simulink model "gm_rampa_vnl"  (R2017a)
settings: Solver=FixedStepDiscrete  StartTime=0.0  StopTime=10.0  FixedStep=0.001  MaxStep=1e-4  RelTol=1e-3
undefined symbols (not defined in the file or in its folder): N
libraries: simulink x2
settings Model: Creator=Windows  LastModifiedBy=Windows
settings DataIOCC: LimitDataPoints=on  SaveOutput=off  SaveTime=off
settings OptimizationCC: BlockReduction=off  ConditionallyExecuteInputs=off  DefaultParameterBehavior=Inlined  LifeSpan=inf
settings DebuggingCC: AlgebraicLoopMsg=error  InheritedTsInSrcMsg=none  SingleTaskRateTransMsg=error  AllowSymbolicDim=off  StrictBusMsg=ErrorOnBusTreatedAsVector  SFUnexpectedBacktrackingDiag=warning  SFNoUnconditionalDefaultTransitionDiag=warning  SFExecutionAtInitializationDiag=none
settings HardwareCC: ProdBitPerPointer=32  ProdBitPerSizeT=32  ProdBitPerPtrDiffT=32  ProdLargestAtomicFloat=None  ProdIntDivRoundTo=Undefined  ProdEndianess=Unspecified  ProdWordSize=32  ProdHWDeviceType=ASIC/FPGA->ASIC/FPGA  TargetBitPerPointer=64  TargetBitPerSizeT=64  TargetBitPerPtrDiffT=64  TargetLongLongMode=on  TargetIntDivRoundTo=Zero  TargetEndianess=LittleEndian  TargetWordSize=64  TargetHWDeviceType=MATLAB Host  ProdEqTarget=off
settings GRTTargetCC: TargetLangStandard=C89/C90 (ANSI)  GeneratePreprocessorConditionals=Disable all
settings ConfigComp: CovScope=ReferencedModels  CovMetricSettings=dw  CovHtmlReporting=on  CovSaveCumulativeToWorkspaceVar=on  CovSaveSingleToWorkspaceVar=on  CovExternalEMLEnable=off  CovSFcnEnable=off

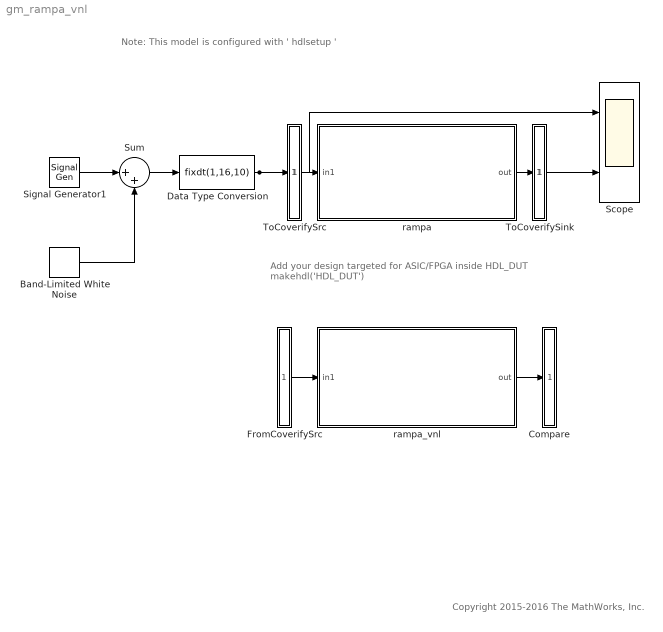
== system gm_rampa_vnl ==
  note: Note: This model is configured with ' hdlsetup '
  note: Add your design targeted for ASIC/FPGA inside HDL_DUT
      | makehdl('HDL_DUT')
  note: Copyright 2015-2016 The MathWorks, Inc.
  Band-Limited White Noise : simulink/Sources/Band-Limited White Noise  Cov=[0.001]  Ts=0.001  seed=[23341]
  Compare : Subsystem
      mask Display: disp('')
  Data Type Conversion : DataTypeConversion  OutDataTypeStr=fixdt(1,16,10)
  FromCoverifySrc : Subsystem
      mask Display: disp('')
  Scope : Scope  NumInputPorts=2
  Signal Generator1 : SignalGenerator  Frequency=2000
  Sum : Sum  Inputs=|++
  ToCoverifySink : Subsystem
      mask Display: disp('')
  ToCoverifySrc : Subsystem
      mask Display: disp('')
  rampa : Subsystem
  rampa_vnl : Subsystem
  wires:
  Data Type Conversion/1 -> Scope/1, ToCoverifySrc/1(in1)
  Signal Generator1/1 -> Sum/1
  Sum/1 -> Data Type Conversion/1
  Band-Limited White Noise/1 -> Sum/2
  ToCoverifySrc/1(out1) -> rampa/1(in1)
  rampa/1(out) -> ToCoverifySink/1(in1)
  ToCoverifySink/1(out1) -> Scope/2
  FromCoverifySrc/1(out1) -> rampa_vnl/1(in1)
  rampa_vnl/1(out) -> Compare/1(in1)

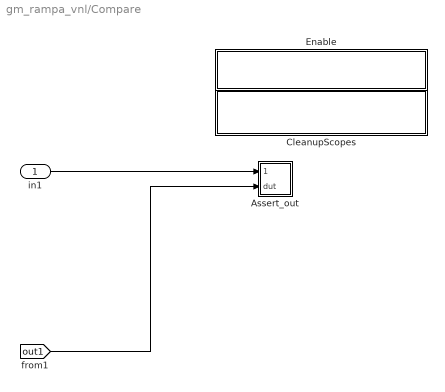
== system gm_rampa_vnl/Compare ==
  in1 : Inport
  Assert_out : Subsystem
  CleanupScopes : Subsystem
      settings: OpenFcn=|
      | blkName = gcb; %self block
      | idx = regexp(blkName, '/CleanupScopes$', 'once');
      | blkParent = blkName(1:idx-1);
      | blks=find_system(blkParent, 'LookUnderMasks', 'all','blocktype', 'Scope');
      | for itr = 1:length(blks)
      | 	 hScopeCfg = get_param(blks{itr},'ScopeConfiguration');
      | 	 hScopeCfg.Visible = ~ hScopeCfg.Visible;
      | end
      | drawnow;
      mask Display: fprintf(message('hdlcoder:cosim:vnl_dblclick').getString());
  Enable : Subsystem
      settings: OpenFcn=|
      | blkName = gcb;
      | idx = regexp(blkName, '/Enable$', 'once');
      | blkParent = blkName(1:idx-1);
      | blks=find_system(blkParent, 'LookUnderMasks', 'all','blocktype', 'Assertion');
      | e = get_param(blks{1}, 'Enabled');
      | if strcmp(e, 'on'), f= 'off';, else, f = 'on';, end
      | for ii=1:length(blks), set_param(blks{ii}, 'Enabled', f);, end
      | set_param(gcb, 'MaskDisplay',['fprintf(message(''hdlcoder:cosim:vnl_dblclick_assertions'',','''',upper(e),'''',').getString())']);
      mask Display: fprintf(message('hdlcoder:cosim:vnl_dblclick_assertions','OFF').getString());
  wires:
  in1/1 -> Assert_out/1(cosim)
  [out1] -> Assert_out/2(dut)

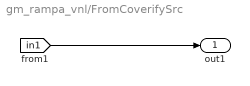
== system gm_rampa_vnl/FromCoverifySrc ==
  out1 : Outport
  wires:
  [in1] -> out1/1

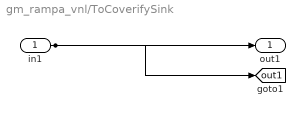
== system gm_rampa_vnl/ToCoverifySink ==
  in1 : Inport
  out1 : Outport
  tag scope: out1=global
  wires:
  in1/1 -> out1/1, [out1]

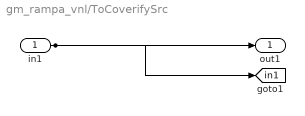
== system gm_rampa_vnl/ToCoverifySrc ==
  in1 : Inport
  out1 : Outport
  tag scope: in1=global
  wires:
  in1/1 -> out1/1, [in1]

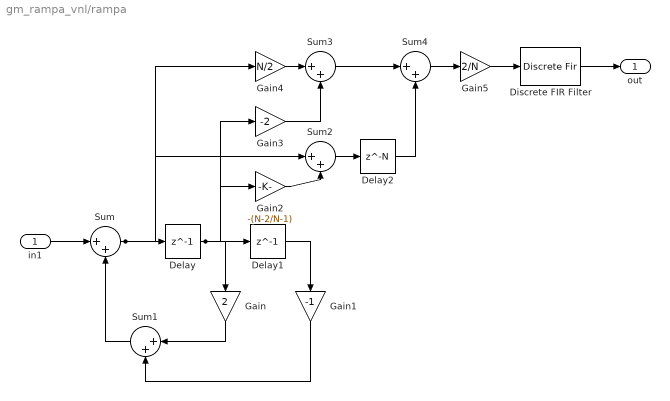
== system gm_rampa_vnl/rampa ==
  in1 : Inport  OutDataTypeStr=fixdt(1, 16, 10)  SampleTime=0
  Delay : Delay  DelayLength=1
  Delay1 : Delay  DelayLength=1
  Delay2 : Delay  DelayLength=N
  Discrete FIR Filter : DiscreteFir  Coefficients=[0.1095 0.1047 0.1000 0.0952 0.0904 0.0857 0.0809 0.0761 0.0714 0.0666 0.0619 0.0571 0.0523 0.0476 0.0428 0.0380 0.0333 0.0285 0.0238 0.0190 0.0142 0.0095 0.0047 0 -0.0047 -0.0095 -0.0142 -0.0190 -0.0238 -0.0285 -0.0333 -0.0380 -0.0428 -0.0476 -0.0523]  CoefDataTypeStr=fixdt(1,16,10)  ProductDataTypeStr=fixdt(1,16,10)  AccumDataTypeStr=fixdt(1,16,10)  OutDataTypeStr=fixdt(1,16,10)
  Gain : Gain  Gain=2
  Gain1 : Gain  Gain=-1
  Gain2 : Gain  Gain=-(N-2/N-1)
  Gain3 : Gain  Gain=-2
  Gain4 : Gain  Gain=N/2
  Gain5 : Gain  Gain=2/N
  Sum{,1..4} (5 alike) : Sum  Inputs=|++  AccumDataTypeStr=fixdt(1,16,10)  OutDataTypeStr=fixdt(1,16,10)
  out : Outport  OutDataTypeStr=fixdt(1,16,10)
  wires:
  Sum4/1 -> Gain5/1
  Sum3/1 -> Sum4/1
  Sum2/1 -> Delay2/1
  Sum1/1 -> Sum/2
  Sum/1 -> Delay/1, Gain4/1, Sum2/1
  Gain5/1 -> Discrete FIR Filter/1
  Gain4/1 -> Sum3/1
  Gain3/1 -> Sum3/2
  Gain2/1 -> Sum2/2
  Gain1/1 -> Sum1/2
  Gain/1 -> Sum1/1
  Discrete FIR Filter/1 -> out/1
  Delay2/1 -> Sum4/2
  Delay1/1 -> Gain1/1
  Delay/1 -> Delay1/1, Gain/1, Gain2/1, Gain3/1
  in1/1 -> Sum/1

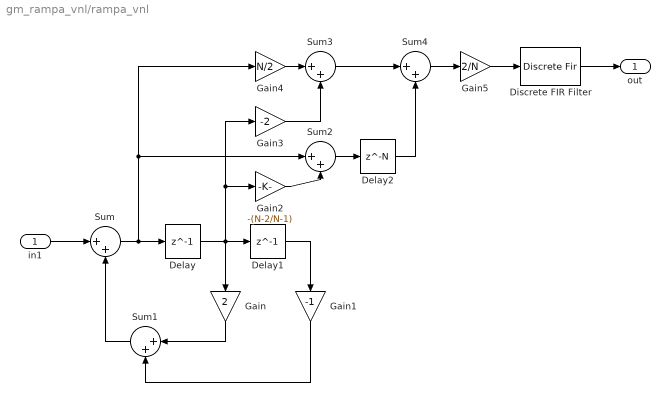
== system gm_rampa_vnl/rampa_vnl ==
  in1 : Inport
  Delay : Delay  DelayLength=1
  Delay1 : Delay  DelayLength=1
  Delay2 : Delay  DelayLength=N
  Discrete FIR Filter : DiscreteFir  Coefficients=[0.1095 0.1047 0.1000 0.0952 0.0904 0.0857 0.0809 0.0761 0.0714 0.0666 0.0619 0.0571 0.0523 0.0476 0.0428 0.0380 0.0333 0.0285 0.0238 0.0190 0.0142 0.0095 0.0047 0 -0.0047 -0.0095 -0.0142 -0.0190 -0.0238 -0.0285 -0.0333 -0.0380 -0.0428 -0.0476 -0.0523]  CoefDataTypeStr=fixdt(1,16,10)  ProductDataTypeStr=fixdt(1,16,10)  AccumDataTypeStr=fixdt(1,16,10)  OutDataTypeStr=fixdt(1,16,10)
  Gain : Gain  Gain=2
  Gain1 : Gain  Gain=-1
  Gain2 : Gain  Gain=-(N-2/N-1)
  Gain3 : Gain  Gain=-2
  Gain4 : Gain  Gain=N/2
  Gain5 : Gain  Gain=2/N
  Sum{,1..4} (5 alike) : Sum  Inputs=|++  AccumDataTypeStr=fixdt(1,16,10)  OutDataTypeStr=fixdt(1,16,10)
  out : Outport  OutDataTypeStr=fixdt(1,16,10)
  wires:
  Discrete FIR Filter/1 -> out/1
  Gain5/1 -> Discrete FIR Filter/1
  Sum4/1 -> Gain5/1
  Delay2/1 -> Sum4/2
  Sum3/1 -> Sum4/1
  Sum2/1 -> Delay2/1
  Gain3/1 -> Sum3/2
  Gain4/1 -> Sum3/1
  Gain2/1 -> Sum2/2
  Sum1/1 -> Sum/2
  Gain1/1 -> Sum1/2
  Gain/1 -> Sum1/1
  Delay1/1 -> Gain1/1
  Delay/1 -> Delay1/1, Gain/1, Gain2/1, Gain3/1
  Sum/1 -> Delay/1, Sum2/1, Gain4/1
  in1/1 -> Sum/1

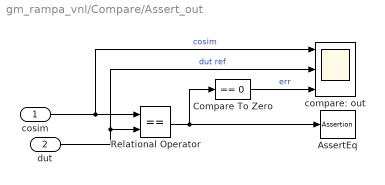
== system gm_rampa_vnl/Compare/Assert_out ==
  cosim : Inport
  dut : Inport  Port=2
  AssertEq : Assertion  StopWhenAssertionFail=off
  Compare To Zero : simulink/Logic and Bit Operations/Compare To Zero  relop===  OutDataTypeStr=boolean
  Relational Operator : RelationalOperator  Operator===  OutDataTypeStr=boolean  RndMeth=Nearest
  compare: out : Scope  NumInputPorts=3
  wires:
  Compare To Zero/1 -> compare: out/3  "err"
  Relational Operator/1 -> Compare To Zero/1, AssertEq/1
  cosim/1 -> compare: out/1, Relational Operator/1  "cosim"
  dut/1 -> compare: out/2, Relational Operator/2  "dut ref"

== system gm_rampa_vnl/Compare/CleanupScopes ==

== system gm_rampa_vnl/Compare/Enable ==
